simulink subsystem "Day1_Scenario_3_4"  (R2024a)
settings: Solver=VariableStepAuto  StartTime=0.0  StopTime=10.0  RelTol=1e-3
libraries: CarMaker4SL x3
settings Model: Creator=junhyung.cha  LastModifiedBy=User

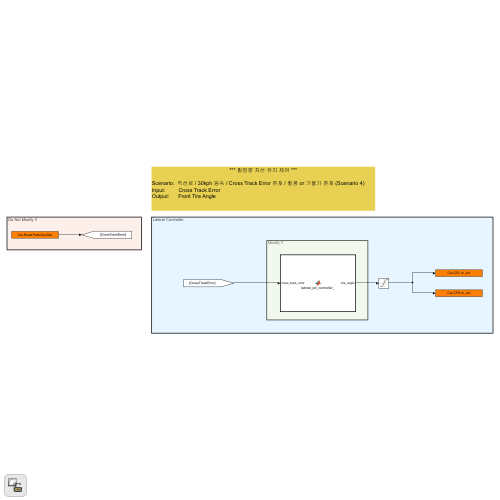
[thumbnail: Simulink's stored preview of the top-level diagram]
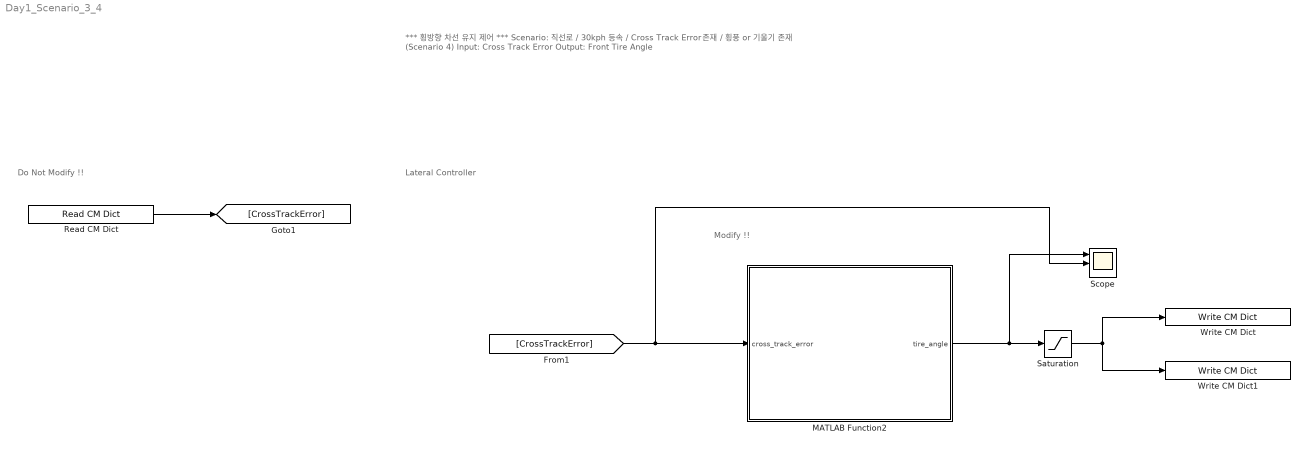
== system Day1_Scenario_3_4 ==
  note: Do Not Modify !!
  note: Modify !!
  note: Lateral Controller
  note: *** 횡방향 차선 유지 제어 ***
      |
      | Scenario: 직선로 / 30kph 등속 / Cross Track Error 존재 / 횡풍 or 기울기 존재 (Scenario 4)
      | Input: Cross Track Error
      | Output: Front Tire Angle
  MATLAB Function2 : MATLAB Function  TreatAsAtomicUnit=on
  Read CM Dict : CarMaker4SL/Read CM Dict  xname=Car.Road.Path.DevDist  xsync=off  xstime=Inherited
  Saturation : Saturate  UpperLimit=2  LowerLimit=-2
  Scope : Scope  NumInputPorts=3
  Write CM Dict : CarMaker4SL/Write CM Dict  xname=Car.CFL.rz_ext  xsync=off
  Write CM Dict1 : CarMaker4SL/Write CM Dict  xname=Car.CFR.rz_ext  xsync=off
  wires:
  Read CM Dict/1 -> [CrossTrackError]
  MATLAB Function2/1(tire_angle) -> Saturation/1, Scope/1
  [CrossTrackError] -> MATLAB Function2/1(cross_track_error), Scope/2
  Saturation/1 -> Write CM Dict/1, Write CM Dict1/1

== matlab function Day1_Scenario_3_4/MATLAB Function2 ==
  settings: updateMethod=DISCRETE  sampleTime=0.05
  data: cross_track_error input; tire_angle output
% 1. 이전 오차 기억
% 2. 현재 오차와의 차이를 통해 미분항 계산
% 3. 현재 오차와 미분항을 기반으로 조향각 계산
% 4. 현재 오차를 저장해 다음에 사용할 준비

function tire_angle = lateral_pd_controller_(cross_track_error)

persistent prev_error % 이전 오차
persistent initialized % 시작 여부

dt = 0.001;

Kp = 0.31;
Kd = 0.0031;

if isempty(initialized)
    prev_error = 0;
    initialized = true;
end

derivative = (cross_track_error - prev_error) / dt;

tire_angle = -Kp * cross_track_error - Kd * derivative;


prev_error = cross_track_error;
